simulink model "lab4_2"  (R2020a)
settings: Solver=VariableStepAuto  StartTime=0.0  StopTime=20.0  RelTol=10e-10  AbsTol=10e-10
values from neighbouring files (symbols this model uses):
  d_bar = (Ra/Kt)*(tau_1)    (= 3)    [Lab4.m]    (also in lab4.m)
  Kaw = 1/0.21    (= 4.7619047619)    [Lab4.m]
  thetades = pi/2    (= 1.57079632679)    [Lab4.m]    (also in lab4.m)
  Ti = 10/Wcp_C1G    [Lab4.m]    (also in lab4.m)
  Vlim = 5    [Lab4.m]    (also in lab4.m)
libraries: cstblocks x2
settings Model: Creator=paulosga  LastModifiedBy=paulosga

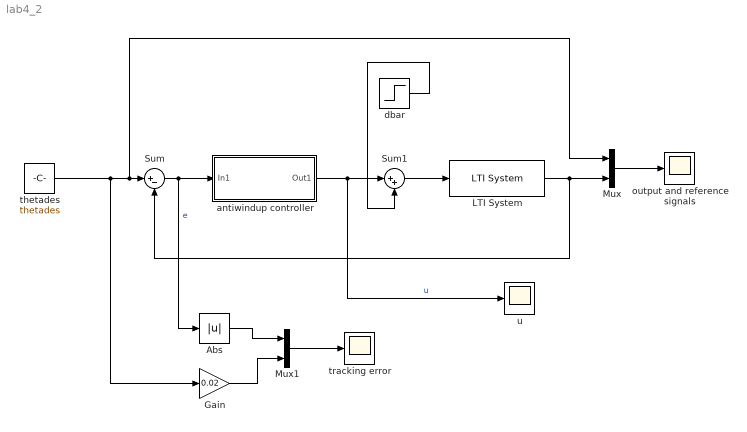
== system lab4_2 ==
  Abs : Abs
  Gain : Gain  Gain=0.02
  LTI System : cstblocks/LTI System  sys=G  IC=[]
  Mux : Mux  Inputs=2
  Mux1 : Mux  Inputs=2
  Sum : Sum  Inputs=|+-
  Sum1 : Sum  Inputs=|++
  antiwindup controller : Subsystem
  dbar : Step  Time=5  After=d_bar  SampleTime=0
  output and reference signals : Scope
  thetades : Constant  Value=thetades
  tracking error : Scope
  u : Scope
  wires:
  Mux1/1 -> tracking error/1
  Sum1/1 -> LTI System/1
  Gain/1 -> Mux1/2
  Abs/1 -> Mux1/1
  dbar/1 -> Sum1/2
  antiwindup controller/1(Out1) -> u/1, Sum1/1  "u"
  Mux/1 -> output and reference signals/1
  thetades/1 -> Gain/1, Mux/1, Sum/1
  LTI System/1 -> Mux/2, Sum/2
  Sum/1 -> antiwindup controller/1(In1), Abs/1  "e"

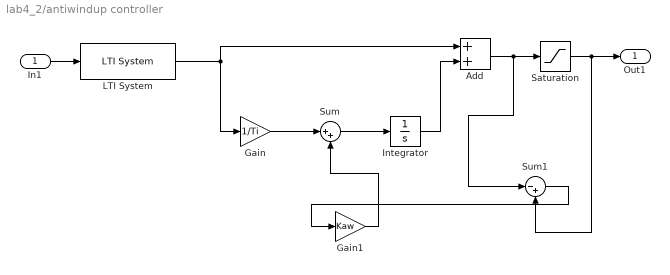
== system lab4_2/antiwindup controller ==
  In1 : Inport
  Add : Sum
  Gain : Gain  Gain=1/Ti
  Gain1 : Gain  Gain=Kaw
  Integrator : Integrator
  LTI System : cstblocks/LTI System  sys=C1  IC=[]
  Saturation : Saturate  UpperLimit=Vlim  LowerLimit=-Vlim
  Sum : Sum  Inputs=|++
  Sum1 : Sum  Inputs=|-+
  Out1 : Outport
  wires:
  In1/1 -> LTI System/1
  LTI System/1 -> Gain/1, Add/1
  Gain/1 -> Sum/1
  Sum/1 -> Integrator/1
  Integrator/1 -> Add/2
  Add/1 -> Sum1/1, Saturation/1
  Sum1/1 -> Gain1/1
  Saturation/1 -> Sum1/2, Out1/1
  Gain1/1 -> Sum/2
